simulink model "KUKA_EE_Controller_v4"  (R2021b)
settings: Solver=ode4  StartTime=0.0  StopTime=100  FixedStep=0.01  RelTol=1e-3
InitFcn:
  | %rho_0t=[0.29;0.29;0.29]; %m
  | %V_0t=[-0.001;-0.001;0];%[-0.0005;-0.0005;0];
  | %w_t=[0;0;-0.002];
  | 
  | 
  | %rho_0t=[0.3;0.3;0.2]; %m
  | %V_0t=[-0.001;-0.001;0];%[-0.0005;-0.0005;0];
  | %w_t=[0;0;-0.001];
values from neighbouring files (symbols this model uses):
  g_cm = zeros(4,4,n)    [Main.m]
  Im = zeros(3,3,n)    [Main.m]
  iota0 = eye(6,6)    [Internal_KUKA_Main.m]    (also in KUKA_Main.m; Main.m)
  K_d = 10*[1.3*eye(3) zeros(3);zeros(3) 0.8*eye(3)]    [Initiate_FQ.m]    (also in Internal_KUKA_Main.m = 200*[0.7*eye(3) zeros(3);zeros(3) 0.5*eye(3)]; KUKA_Main.m = [0.7*eye(3) zeros(3);zeros(3) 0.5*eye(3)]; Main.m = eye(6))
  K_i = 5*[0.1*eye(3) zeros(3);zeros(3) 0.01*eye(3)]    [Initiate_FQ.m]    (also in Internal_KUKA_Main.m = 200*[0.01*eye(3) zeros(3);zeros(3) 0.001*eye(3)]; KUKA_Main.m = [0.01*eye(3) zeros(3);zeros(3) 0.001*eye(3)]; Main.m = eye(6))
  K_p = 50*[0.1 0 0 0 0 0;0 0.1 0 0 0 0; 0 0 0.1 0 0 0; 0 0 0 0.01 0 0 ... (first row only)    [Initiate_FQ.m]    (also in Internal_KUKA_Main.m = 200*[0.1 0 0 0 0 0;0 0.1 0 0 0 0; 0 0 0.1 0 0 0; 0 0 0 0.01 ; KUKA_Main.m = [0.1 0 0 0 0 0;0 0.1 0 0 0 0; 0 0 0.1 0 0 0; 0 0 0 0.01 0 0; Main.m = eye(6))
  K_w = 20*eye(7)    [Initiate_FQ.m]
  K_wd = 1*eye(7)    [Initiate_FQ.m]
  M0 = M_temp.M0.data(:,:,1)    [Initiate_FQ.m]    (also in Internal_KUKA_Main.m; KUKA_Main.m; Main.m = simplify(transpose(robot.vehicle.iota_0)*robot.vehicle.M_fra)
  m0 = robot.Bodies{1,n+1}.Mass    [Internal_KUKA_Main.m]    (also in KUKA_Main.m; Main.m = 100)
  M0m = M_temp.M0m.data(:,:,1)    [Initiate_FQ.m]    (also in Internal_KUKA_Main.m; KUKA_Main.m; Main.m = simplify(transpose(robot.vehicle.iota_0)*transpose(Lm0)*diag)
  M_t = [eye(3)*mt zeros(3); zeros(3) eye(3)*0.416667]    [Initiate_FQ.m]    (also in Internal_KUKA_Main.m = [eye(3)*mt zeros(3); zeros(3) eye(3)*80]; KUKA_Main.m = [eye(3)*mt zeros(3); zeros(3) eye(3)*80]; Main.m = [eye(3)*mt zeros(3); zeros(3) eye(3)*416.667])
  Mm = simplify(transpose(Xi_m)*transpose(Lm)*diagM*Lm*Xi_m)    [Internal_KUKA_Main.m]    (also in KUKA_Main.m; Main.m)
  mm = zeros(1,n)    [Internal_KUKA_Main.m]    (also in KUKA_Main.m; Main.m = [2 2 0])
  mu = -10.*P0    [Initiate_FQ.m]    (also in Internal_KUKA_Main.m = P; KUKA_Main.m = P; Main.m = zeros(6,1)')
  mu_t = -10.*M_t*[V_0t;w_t]    [Initiate_FQ.m]    (also in Internal_KUKA_Main.m = M_t*[V_0t;w_t]; KUKA_Main.m = M_t*[V_0t;w_t]; Main.m = zeros(6,1)')
  q_dot_m = 0.01*q_dot_m    [Initiate_FQ.m]    (also in Internal_KUKA_Main.m = [qdot1;qdot2;qdot3;qdot4;qdot5;qdot6;qdot7]; KUKA_Main.m = [qdot1;qdot2;qdot3;qdot4;qdot5;qdot6;qdot7]; Main.m = [0;0;0;0;0;0;0]; sendJointTorques.m = fread(t, 7, 'double'))
  q_m = [0.2;1.2;0.3;1.8;0.5;1.3;0.6]    [Initiate_FQ.m]    (also in Internal_KUKA_Main.m = [q_m1;q_m2;q_m3;q_m4;q_m5;q_m6;q_m7]; KUKA_Main.m = [q_m1;q_m2;q_m3;q_m4;q_m5;q_m6;q_m7]; Main.m = [0;0;0;0;0;0;0]; sendJointTorques.m = fread(t, 7, 'double'))
  rho_0t = [0;0;0.2]    [Initiate_FQ.m]    (also in Internal_KUKA_Main.m = [0.24;0.26;0.25]; KUKA_Main.m = [0.23;0.27;0.26])
  sc_size = 0    [Internal_KUKA_Main.m]    (also in KUKA_Main.m = 1)
  V_0t = -[-0.0005;-0.0005;0]    [Initiate_FQ.m]    (also in Internal_KUKA_Main.m = [-0.01;-0.01;0]; KUKA_Main.m = [-0.002;-0.002;0])
  V_I0 = 0.01*V_I0    [Initiate_FQ.m]    (also in Internal_KUKA_Main.m = [0;0;0;0;0;0]; KUKA_Main.m = [0;0;0;0;0;0]; Main.m = [0;0;0;0;0;0])
  X = [0 -x(3) x(2) ; x(3) 0 -x(1) ; -x(2) x(1) 0 ]    [skewsym.m]
  Xi_m = Xi_m(1:robot.n*6,1:robot.n)    [Internal_KUKA_Main.m]    (also in KUKA_Main.m; Main.m)
  Xi_m_matrix = zeros(6*n,n)    [Internal_KUKA_Main.m]    (also in KUKA_Main.m; Main.m)
undefined symbols (not defined in the file or in its folder): g_cm0, I0, Ie, m0_frak, m_diag, me, Y, Z
libraries: sm_lib x174, nesl_utility x172, robotcorelib x7
(part 8 of 8)

== matlab function KUKA_EE_Controller_v4/Inverse Dynamics3/C_hat1/AMA_partial ==
  data: q_m input; AMA_partial output; M0 input; A input; A_partial input; V input; M0_partial input
function AMA_partial = AMA_partial(q_m,M0,A,A_partial,V,M0_partial)
% Calculates the C_hat_m matrix from base pose and arm joint angles

n=length(q_m);
b=length(V);

% find the temp intermediate term
AMA_partial=zeros(n,n,n);
for i=1:n
    AMA_partial(1:n,1:n,i)=transpose(A_partial(1:end,1:end,i))*M0*A+transpose(A)*M0_partial(1:end,1:end,i)*A+transpose(A)*M0*A_partial(1:end,1:end,i); %calcualte the derivative of not-augmented arm mass matrix from equation 121 of TRO paper
end

== matlab function KUKA_EE_Controller_v4/Inverse Dynamics3/C_hat1/A_partial ==
  data: q_m input; A_partial output; M0 input; M0_partial input; M0m_partial input; M0m input; V input
function A_partial = A_partial(q_m,M0,M0_partial,M0m_partial,M0m,V)
% Calculates the C_hat_m matrix from base pose and arm joint angles

n=length(q_m);
b=length(V);

% Find partial of connection A to each joint angle
A_partial=zeros(b,n,n);

temp1=zeros(b,n);
temp2=zeros(b,n);
temp3=zeros(b,n);

for i=1:n
    temp1=M0\M0_partial(1:end,1:end,i);
    temp2=M0\M0m;
    temp3=M0\M0m_partial(1:end,1:end,i);
    A_partial(1:b,1:n,i)=-temp1*temp2+temp3; % Equation 122
end

== matlab function KUKA_EE_Controller_v4/Dynamic Parameters/ 1 ==
  data: q_m input; L0 output; Lm0 output; Lm output; Xi_m input
function [L0,Lm0,Lm] =L_calculator(q_m,Xi_m)
% Calculates the time-dependent L matrix
n=length(q_m);
L=zeros(6*(n+1),6*(n+1));
% Compute M_frak for ith body
% Calculate L matrix
for i=1:n+1
    for j=1:n+1
        if i>j
            Ad_temp=eye(6);
            for k=j:i-1
                Ad_temp=Adjoint(g_Matrix(-Xi_m(:,k),q_m(k)))*Ad_temp;
            end
            L(6*(i-1)+1:6*(i-1)+6,6*(j-1)+1:6*(j-1)+6)=Ad_temp;
        elseif i==j
            L(6*(i-1)+1:6*(i-1)+6,6*(j-1)+1:6*(j-1)+6)=eye(6);
        elseif i<j
            L(6*(i-1)+1:6*(i-1)+6,6*(j-1)+1:6*(j-1)+6)=zeros(6);
        end
    end
end

L0=L(1:6,1:6);
Lm0=L(7:end,1:6);
Lm=L(7:end,7:end);

end

== matlab function KUKA_EE_Controller_v4/Inverse Dynamics3/C_hat1/C_hat ==
  data: q_m input; Mm_hat_partial input; q_dot_m input; C_hat output
function C_hat = C_hat(q_m, Mm_hat_partial,q_dot_m)
% Calculates the C_hat_m matrix from base pose and arm joint angles

n=length(q_m);


% Calculate C_hat matrix
C_temp1=zeros(n,n);
C_temp2=zeros(n,n);
C_hat=zeros(n,n);
for i=1:n
    C_temp1=C_temp1+squeeze(Mm_hat_partial(1:n,1:n,i)).*q_dot_m(i); % nxn by scalar
    C_temp2(i,1:n)=0.5*transpose(q_dot_m)*squeeze(Mm_hat_partial(1:n,1:n,i)); %1xn by nxn 
end

C_hat=C_temp1-C_temp2;

== matlab function KUKA_EE_Controller_v4/Inverse Dynamics3/C_hat1/Lm_partials/Lm0partial ==
  data: q_m input; Lm0_partial output; Xi_m input; iota0 input
function Lm0_partial = Lm0_partial(q_m,Xi_m,iota0)
% Calculates the C_hat_m matrix from base pose and arm joint angles

n=length(q_m);

% Find partial of Lm to joint angles
Lm0_partial=zeros(6*n,6,n); % 6nx6xn
for i=1:n
    for j=1:n
        Lm0_partial(6*(j-1)+1:6*j,1:6,i)=Ad_partial(j,1,i,Xi_m,q_m,iota0); % equation 114 of TRO paper
    end
end

%%%%%%%%%%%%%%%%%%%%%%%%%%%%%%%%%%%%%%%%%%%%%%%%%%%%%%%%%%%%% MUST BE
%%%%%%%%%%%%%%%%%%%%%%%%%%%%%%%%%%%%%%%%%%%%%%%%%%%%%%%%%%%%% CHECKED

== matlab function KUKA_EE_Controller_v4/Inverse Dynamics3/C_hat1/Lm_partials/Lmpartial ==
  data: q_m input; Lm_partial output; Xi_m input; iota0 input
function Lm_partial  = Lm_partial(q_m,Xi_m,iota0)
% Calculates the C_hat_m matrix from base pose and arm joint angles

n=length(q_m);

% Find partial of Lm0 to joint angles
Lm_partial=zeros(6*n,6*n,n); % 6nx6xn
for i=1:n
    Lm_partial(:,:,i)=zeros(6*n,6*n);
    for j=2:n
        for k=2:n
            if j>i && i>=k
                Lm_partial(6*(j-1)+1:6*j,6*(k-2)+1:6*(k-1),i)=Ad_partial(j,k,i,Xi_m,q_m,iota0); % equation 81 of TRO paper
            elseif i==j && i>=k
                Lm_partial(6*(j-1)+1:6*j,6*(k-2)+1:6*(k-1),i)=Ad_partial(j,k,i,Xi_m,q_m,iota0); % equation 81 of TRO paper
            else
                Lm_partial(6*(j-1)+1:6*(j-1)+6,6*(k-2)+1:6*(k-2)+6,i)=zeros(6,6);
            end

        end
    end
end

== matlab function KUKA_EE_Controller_v4/Inverse Dynamics3/C_hat1/M_partials/ M0partial ==
  data: q_m input; M0_partial output; Lm0 input; V input; iota0 input; diag_Mm input; Lm0_partial input
function M0_partial = M0_partial(q_m,Lm0,V,iota0,diag_Mm,Lm0_partial)
% Calculates the C_hat_m matrix from base pose and arm joint angles

n=length(q_m);
b=length(V);

% Find partial of M0 to joint angles
M0_partial=zeros(b,b,n); %initiate
for i=1:n
    temp1=transpose(Lm0_partial(1:end,1:end,i))*diag_Mm*Lm0;
    temp2=transpose(Lm0)*diag_Mm*Lm0_partial(1:end,1:end,i);
    M0_partial(1:b,1:b,i)= iota0'*(temp1+temp2)*iota0; %6x6 %equation 117 of TRO
end

== matlab function KUKA_EE_Controller_v4/Inverse Dynamics3/C_hat1/M_partials/M0mpartial ==
  data: q_m input; M0m_partial output; V input; Lm input; Lm0 input; iota0 input; diag_Mm input; Lm0_partial input; Lm_partial input; Xi_m_matrix input
function M0m_partial = M0m_partial(q_m,V,Lm,Lm0,iota0,diag_Mm,Lm0_partial,Lm_partial, Xi_m_matrix)
% Calculates the C_hat_m matrix from base pose and arm joint angles

n=length(q_m);
b=length(V);

% Find partial of M0m to joint angles
M0m_partial=zeros(b,n,n);
for i=1:n
    temp1=transpose(Lm0_partial(1:end,1:end,i))*diag_Mm*Lm;
    temp2=transpose(Lm0)*diag_Mm*Lm_partial(1:end,1:end,i);
    M0m_partial(1:b,1:n,i)= iota0'*(temp1+temp2)*Xi_m_matrix; % equation 118 of TRO paper
end

== matlab function KUKA_EE_Controller_v4/Inverse Dynamics3/C_hat1/M_partials/Mmpartial ==
  data: q_m input; Mm_partial output; Xi_m_matrix input; Lm input; diag_Mm input; Lm_partial input
function Mm_partial = Mm_partial(q_m,Xi_m_matrix,Lm,diag_Mm,Lm_partial)
% Calculates the C_hat_m matrix from base pose and arm joint angles

n=length(q_m);

% find the non-generalized arm mass matrix'x derivative to joint angles
Mm_partial=zeros(n,n,n);
for i=1:n
    temp=   transpose(Lm_partial(1:6*n,1:6*n,i))*diag_Mm*Lm  +   transpose(Lm)*diag_Mm*Lm_partial(1:6*n,1:6*n,i);
    Mm_partial(1:n,1:n,i)=transpose(Xi_m_matrix)*temp*Xi_m_matrix; %calcualte the derivative of not-augmented arm mass matrix from equation 120 of TRO paper
end

== matlab function KUKA_EE_Controller_v4/Inverse Dynamics3/C_hat1/Mm_hat_partial ==
  data: q_m input; AMA_partial input; Mm_hat_partial output; Mm_partial input
function Mm_hat_partial = Mm_hat_partial(q_m, AMA_partial, Mm_partial)
% Calculates the C_hat_m matrix from base pose and arm joint angles

n=length(q_m);

% find the generalized arm mass matrix'x derivative to joint angles
Mm_hat_partial=zeros(n,n,n);
for i=1:n
    Mm_hat_partial(1:n,1:n,i)=Mm_partial(1:n,1:n,i)-AMA_partial(1:n,1:n,i); %calcualte the derivative of augmented arm mass matrix from equation 119 of TRO paper
end

== matlab function KUKA_EE_Controller_v4/Inverse Dynamics3/N_hat1/N_hat ==
  data: N_hat_temp output; q_m input; q_dot_m input; A input; V input; P input; M0_partial input; A_partial input; iota0 input; M0 input
function N_hat_temp = N_hat(q_m,q_dot_m,A,V,P,M0_partial, A_partial, iota0, M0)
% Calculates the N_hat_m matrix from base pose and arm joint angles

n=length(q_m);
b=length(V);

%Form N_hat from equation 19 of ACC paper
N_temp1=zeros(n,b); N_temp2=zeros(n,b); N_temp3=zeros(n,b);

for i=1:n
    N_temp1=N_temp1+transpose(squeeze(A_partial(1:b,1:n,i)).*q_dot_m(i)); % transpose of (bxn times 1x1) 
    N_temp2(i,1:b)=transpose(q_dot_m)*transpose(squeeze(A_partial(1:b,1:n,i))); %1xn times nxb
    N_temp3(i,1:b)=0.5*transpose(P)*(M0\M0_partial(1:end,1:end,i))*inv(M0); % 1xb times bxb
end

N_hat_temp=transpose(A)*transpose(adjoint_low(V,iota0))-N_temp1+N_temp2+N_temp3;

== matlab function KUKA_EE_Controller_v4/Space Manipulator2/Q2q ==
  data: Q input; qm output
function qm = Q2q(Q)

qm=quat2eul(Q','XYZ')';

== matlab function KUKA_EE_Controller_v4/Controller/Velocity_error ==
  data: g_I0 input; V_Ie input; U_ff output; V_It input; V_It_dot input
function U_ff = U_ff(g_I0, V_Ie,V_It, V_It_dot)

U_ff=adjoint_low(Adjoint(g_I0)*V_Ie)*Adjoint(inv(g_I0))*V_It+Adjoint(inv(g_I0))*V_It_dot;

== matlab function KUKA_EE_Controller_v4/Space Manipulator2/Q2q1 ==
  data: Q input; qm output
function qm = Q2q(Q)

qm=quat2eul(Q','XYZ')';

== matlab function KUKA_EE_Controller_v4/Inverse Dynamics3/A_dot ==
  data: A_partial input; q_m input; A_dot output
function A_dot = fcn(A_partial, q_m)
n=length(q_m);

A_dot=zeros(6,n);
for i=1:n
    A_dot=A_dot+A_partial(:,:,i).*q_m(i);
end

== matlab function KUKA_EE_Controller_v4/Inverse Dynamics3/C_hat/AMA_partial ==
  data: q_m input; AMA_partial output; M0 input; A input; A_partial input; V input; M0_partial input
function AMA_partial = AMA_partial(q_m,M0,A,A_partial,V,M0_partial)
% Calculates the C_hat_m matrix from base pose and arm joint angles

n=length(q_m);
b=length(V);

% find the temp intermediate term
AMA_partial=zeros(n,n,n);
for i=1:n
    AMA_partial(1:n,1:n,i)=transpose(A_partial(1:end,1:end,i))*M0*A+transpose(A)*M0_partial(1:end,1:end,i)*A+transpose(A)*M0*A_partial(1:end,1:end,i); %calcualte the derivative of not-augmented arm mass matrix from equation 121 of TRO paper
end

== matlab function KUKA_EE_Controller_v4/Inverse Dynamics3/C_hat/A_partial ==
  data: q_m input; A_partial output; M0 input; M0_partial input; M0m_partial input; M0m input; V input
function A_partial = A_partial(q_m,M0,M0_partial,M0m_partial,M0m,V)
% Calculates the C_hat_m matrix from base pose and arm joint angles

n=length(q_m);
b=length(V);

% Find partial of connection A to each joint angle
A_partial=zeros(b,n,n);

temp1=zeros(b,n);
temp2=zeros(b,n);
temp3=zeros(b,n);

for i=1:n
    temp1=M0\(M0_partial(:,:,i));
    temp2=M0\M0m;
    temp3=M0\(M0m_partial(:,:,i));
    A_partial(1:b,1:n,i)=-temp1*temp2+temp3; % Equation 122
end

== matlab function KUKA_EE_Controller_v4/Inverse Dynamics3/C_hat/C_hat1 ==
  data: q_m input; Mm_hat_partial input; q_dot_m input; C_hat output
function C_hat = C_hat(q_m, Mm_hat_partial,q_dot_m)
% Calculates the C_hat_m matrix from base pose and arm joint angles

n=length(q_m);


% Calculate C_hat matrix
C_temp1=zeros(n,n);
C_temp2=zeros(n,n);
C_hat=zeros(n,n);
for i=1:n
    C_temp1=C_temp1+squeeze(Mm_hat_partial(1:n,1:n,i)).*q_dot_m(i); % nxn by scalar
    C_temp2(i,1:n)=0.5*transpose(q_dot_m)*squeeze(Mm_hat_partial(1:n,1:n,i)); %1xn by nxn 
end

C_hat=C_temp1-C_temp2;

== matlab function KUKA_EE_Controller_v4/Inverse Dynamics3/C_hat/Lm_partials/Lm0partial ==
  data: q_m input; Lm0_partial output; Xi_m input; iota0 input
function Lm0_partial = Lm0_partial(q_m,Xi_m,iota0)
% Calculates the C_hat_m matrix from base pose and arm joint angles

n=length(q_m);

% Find partial of Lm to joint angles
Lm0_partial=zeros(6*n,6,n); % 6nx6xn
for i=1:n
    for j=1:n
        Lm0_partial(6*(j-1)+1:6*j,1:6,i)=Ad_partial(j,1,i,Xi_m,q_m,iota0); % equation 114 of TRO paper
    end
end

%%%%%%%%%%%%%%%%%%%%%%%%%%%%%%%%%%%%%%%%%%%%%%%%%%%%%%%%%%%%% MUST BE
%%%%%%%%%%%%%%%%%%%%%%%%%%%%%%%%%%%%%%%%%%%%%%%%%%%%%%%%%%%%% CHECKED

== matlab function KUKA_EE_Controller_v4/Inverse Dynamics3/C_hat/Lm_partials/Lmpartial ==
  data: q_m input; Lm_partial output; Xi_m input; iota0 input
function Lm_partial  = Lm_partial(q_m,Xi_m,iota0)
% Calculates the C_hat_m matrix from base pose and arm joint angles

n=length(q_m);

% Find partial of Lm0 to joint angles
Lm_partial=zeros(6*n,6*n,n); % 6nx6xn
for i=1:n
    Lm_partial(:,:,i)=zeros(6*n,6*n);
    for j=2:n
        for k=2:n
            if j>i && i>=k
                Lm_partial(6*(j-1)+1:6*j,6*(k-2)+1:6*(k-1),i)=Ad_partial(j,k,i,Xi_m,q_m,iota0); % equation 81 of TRO paper
            elseif i==j && i>=k
                Lm_partial(6*(j-1)+1:6*j,6*(k-2)+1:6*(k-1),i)=Ad_partial(j,k,i,Xi_m,q_m,iota0); % equation 81 of TRO paper
            else
                Lm_partial(6*(j-1)+1:6*(j-1)+6,6*(k-2)+1:6*(k-2)+6,i)=zeros(6,6);
            end

        end
    end
end

== matlab function KUKA_EE_Controller_v4/Inverse Dynamics3/C_hat/M_partials/ M0partial ==
  data: q_m input; M0_partial output; Lm0 input; V input; iota0 input; diag_Mm input; Lm0_partial input
function M0_partial = M0_partial(q_m,Lm0,V,iota0,diag_Mm,Lm0_partial)
% Calculates the C_hat_m matrix from base pose and arm joint angles

n=length(q_m);
b=length(V);

% Find partial of M0 to joint angles
M0_partial=zeros(b,b,n); %initiate
for i=1:n
    temp1=transpose(Lm0_partial(1:end,1:end,i))*diag_Mm*Lm0;
    temp2=transpose(Lm0)*diag_Mm*Lm0_partial(1:end,1:end,i);
    M0_partial(1:b,1:b,i)= iota0'*(temp1+temp2)*iota0; %6x6 %equation 117 of TRO
end

== matlab function KUKA_EE_Controller_v4/Inverse Dynamics3/C_hat/M_partials/M0mpartial ==
  data: q_m input; M0m_partial output; V input; Lm input; Lm0 input; iota0 input; diag_Mm input; Lm0_partial input; Lm_partial input; Xi_m_matrix input
function M0m_partial = M0m_partial(q_m,V,Lm,Lm0,iota0,diag_Mm,Lm0_partial,Lm_partial, Xi_m_matrix)
% Calculates the C_hat_m matrix from base pose and arm joint angles

n=length(q_m);
b=length(V);

% Find partial of M0m to joint angles
M0m_partial=zeros(b,n,n);
for i=1:n
    temp1=transpose(Lm0_partial(1:end,1:end,i))*diag_Mm*Lm;
    temp2=transpose(Lm0)*diag_Mm*Lm_partial(1:end,1:end,i);
    M0m_partial(1:b,1:n,i)= iota0'*(temp1+temp2)*Xi_m_matrix; % equation 118 of TRO paper
end

== matlab function KUKA_EE_Controller_v4/Inverse Dynamics3/C_hat/M_partials/Mmpartial ==
  data: q_m input; Mm_partial output; Xi_m_matrix input; Lm input; diag_Mm input; Lm_partial input
function Mm_partial = Mm_partial(q_m,Xi_m_matrix,Lm,diag_Mm,Lm_partial)
% Calculates the C_hat_m matrix from base pose and arm joint angles

n=length(q_m);

% find the non-generalized arm mass matrix'x derivative to joint angles
Mm_partial=zeros(n,n,n);
for i=1:n
    temp=   transpose(Lm_partial(1:6*n,1:6*n,i))*diag_Mm*Lm  +   transpose(Lm)*diag_Mm*Lm_partial(1:6*n,1:6*n,i);
    Mm_partial(1:n,1:n,i)=transpose(Xi_m_matrix)*temp*Xi_m_matrix; %calcualte the derivative of not-augmented arm mass matrix from equation 120 of TRO paper
end

== matlab function KUKA_EE_Controller_v4/Controller/gradient_of_Eg ==
  data: g_te input; Nabla_Eg output
function Nabla_Eg = fcn(g_te)

% Calculate the gradient of the Pose Error Function
p_te=g_te(1:3,4);
R_te=g_te(1:3,1:3);

temp=0.5*(R_te-transpose(R_te));

R_temp=vee3(temp);

Nabla_Eg=[p_te;R_temp];

== matlab function KUKA_EE_Controller_v4/Inverse Dynamics3/C_hat/Mm_hat_partial ==
  data: q_m input; AMA_partial input; Mm_hat_partial output; Mm_partial input
function Mm_hat_partial = Mm_hat_partial(q_m, AMA_partial, Mm_partial)
% Calculates the C_hat_m matrix from base pose and arm joint angles

n=length(q_m);

% find the generalized arm mass matrix'x derivative to joint angles
Mm_hat_partial=zeros(n,n,n);
for i=1:n
    Mm_hat_partial(1:n,1:n,i)=Mm_partial(1:n,1:n,i)-AMA_partial(1:n,1:n,i); %calcualte the derivative of augmented arm mass matrix from equation 119 of TRO paper
end

== matlab function KUKA_EE_Controller_v4/Inverse Dynamics3/Inverse Dynamics/Ad_g_I0_dot ==
  data: g_I0 input; V_I0 input; Ad_g_I0_dot output
function Ad_g_I0_dot = Ad_g_I0_dot(g_I0,V_I0)
% Calculation of F_mu Eq 30 of paper
Ad_g_I0_dot=adjoint_low(V_I0)'*Adjoint(g_I0)';
% adjoint_low(V_I0)*transpose(Adjoint*(g_I0)))

== matlab function KUKA_EE_Controller_v4/Inverse Dynamics3/Inverse Dynamics/Ad_g_I0_dot1 ==
  data: V_t input; Ad_g_It_dot output; g_It input
function Ad_g_It_dot = Ad_g_It_dot(V_t,g_It)
% Calculation of F_mu Eq 30 of paper
Ad_g_It_dot=adjoint_low(V_t)'*Adjoint(g_It)';

== matlab function KUKA_EE_Controller_v4/Inverse Dynamics3/Inverse Dynamics/Ad_g_te_dot ==
  data: V_te input; Ad_g_te_dot output; g_te input
function Ad_g_te_dot = Ad_g_te_dot(V_te,g_te)
% Calculation of F_mu Eq 30 of paper
Ad_g_te_dot=-adjoint_low(V_te)/Adjoint(g_te);

== matlab function KUKA_EE_Controller_v4/Inverse Dynamics3/Inverse Dynamics/FU ==
  data: MmJcross input; F_U output
function F_U = F_U(MmJcross)
F_U=MmJcross;

== matlab function KUKA_EE_Controller_v4/Inverse Dynamics3/Inverse Dynamics/Fm ==
  data: MmJcross input; F_m output; A_dot input; Cm_hat input
function F_m = F_m(MmJcross,A_dot,Cm_hat)
% Calculation of F_mu Eq 30 of paper
F_m=MmJcross*(A_dot)+Cm_hat;

== matlab function KUKA_EE_Controller_v4/Inverse Dynamics3/Inverse Dynamics/Fmu ==
  data: MmJcross input; M0 input; M_0_dot input; g_I0 input; F_mu output; Ad_g_I0_dot input
function F_mu = F_mu(MmJcross,M0,M_0_dot,g_I0,Ad_g_I0_dot)
% Calculation of F_mu Eq 30 of paper
F_mu=-MmJcross*(M0\M_0_dot*inv(M0)*transpose(Adjoint(g_I0))+ ...
    M0\Ad_g_I0_dot);

== matlab function KUKA_EE_Controller_v4/Inverse Dynamics3/Inverse Dynamics/Inverse Dynamics ==
  data: F_mu output; F_t output; F_m output
function [F_mu,F_t,F_m] = fcn()


% n=length(q_m);

%Calculate Mass Matrix block components
% [ M0m Mm]=Mass_Matrix(q_m,Xi_m);

% A=inverse(M0)*M0m; % Mechanical Connection
% Mm_hat=Mm-transpose(A)*M0*A; %augmented manipulator mass matrix
% V=inverse(M0)*(mu-transpose(A)*q_dot_m); %Spacecraft Velocity

% The augmented Jacobian
% J_aug = J_em-J_e0*A;

% for i=1:n
%     for j=1:n
%         Cm_hat=
%     end
% end 

% Find A_dot thru finding partial of connection A to each joint angle
% A_partial=zeros(6,n,n);
% A_dot=zeros(6,n);
% for i=1:n
%     A_partial(6,n,i)=inverse(M0)*M0_partial(1:6,1:6,i)*inverse(M0)*M0m+inverse(M0)*M0m_partial(6,n,i); % Equation 122
%     A_dot(6,n)=A_dot+A_partial(6,n,i).*q_dot_m(i);
% end


% inverse or moore-penrose inverse of the augmented J2 Jacobian matrix
% if rank(J_aug)==size(J2(1,:))
%     J_inv=inverse(J2);
% else
%     J_inv=pinv(J2);
% end

% MJ_inv=-Mm_hat*J_cross;

% J_em_dot=J_em_dot;
% J_e0_dot=J_e0_dot;

% Form the eventual feedback transformation terms
% F_U=MmJcross; %done
% F_mu=MmJcross*(J_e0_dot*inverse(M0)*transpose(Adjoint*(g_I0))- ...
%     J_e0*inverse(M0)*M_0_dot*inverse(M0)*transpose(Adjoint*(g_I0))+ ...
%     J_e0*inverse(M0)*adjoint_low(inverse(M0*transpose(Adjoint(g_I0))*mu)-A*q_dot_m)); 
% F_t=MmJcross*();
% F_m=MmJcross*(J_em_dot-J_e0_dot*A-J_e0*A_dot)+Cm_hat;

== matlab function KUKA_EE_Controller_v4/Controller/Kinematics/g_te ==
  data: g_Ie input; g_It input; g_te output
function g_te = relative_pose(g_Ie, g_It)
% Calculates the relative pose of end-effector to target from the absolute
% poses of the end-effector and the target
g_te = inverse(g_It)*g_Ie;

== matlab function KUKA_EE_Controller_v4/Inverse Dynamics3/Inverse Dynamics/MATLAB Function3 ==
  data: MmJcross input; g_te input; F_t output; g_It input; Mt input; Ad_gte_dot input; Ad_gIt_dot input
function F_t = F_t(MmJcross,g_te,g_It,Mt,Ad_gte_dot,Ad_gIt_dot)
% Calculation of F_mu Eq 30 of paper
F_t=-MmJcross*(Ad_gte_dot/Mt*Adjoint(g_It)'+Adjoint(g_te)\(Mt\Ad_gIt_dot));

% F_t=MmJcross*(-adjoint_low(V_te)/Adjoint(g_te)/Adjoint(g_tt)/M_t/Adjoint(g_It)'+...
%     Adjoint()\); 

% J_e0_dot*inverse(M0)*transpose(Adjoint*(g_I0))- ...
%     J_e0*inverse(M0)*M_0_dot*inverse(M0)*transpose(Adjoint*(g_I0))+ ...
%     J_e0*inverse(M0)*adjoint_low(inverse(M0*transpose(Adjoint(g_I0))*mu)-A*q_dot_m)
%     Ad_g_te_dot

== matlab function KUKA_EE_Controller_v4/Inverse Dynamics3/Inverse Dynamics/MmJcross ==
  data: Mm_hat input; MmJcross output; A input
function MmJcross = MmJcross(Mm_hat, A)

JJ=-A;

% MmJcross = Mm_hat*pinv(JJ);
MmJcross = Mm_hat*pinv(JJ);%,10^(-3)

== matlab function KUKA_EE_Controller_v4/Inverse Dynamics3/Inverse Dynamics/Mm_hat ==
  data: M0 input; Mm_hat output; Mm input; A input
function Mm_hat = Mm_hat(M0,Mm,A)

Mm_hat=Mm-A'*M0*A;

== matlab function KUKA_EE_Controller_v4/Inverse Dynamics3/M0_dot ==
  data: M0_partial input; q_m input; M0_dot output
function M0_dot = fcn(M0_partial, q_m)
n=length(q_m);

M0_dot=zeros(6,6);
for i=1:n
    M0_dot=M0_dot+M0_partial(:,:,i).*q_m(i);
end

== matlab function KUKA_EE_Controller_v4/Inverse Dynamics3/N_hat/N_hat ==
  data: N_hat_temp output; q_m input; q_dot_m input; A input; V input; P input; M0_partial input; A_partial input; iota0 input; M0 input
function N_hat_temp = N_hat(q_m,q_dot_m,A,V,P,M0_partial, A_partial, iota0, M0)
% Calculates the N_hat_m matrix from base pose and arm joint angles

n=length(q_m);
b=length(V);

%Form N_hat from equation 19 of ACC paper
N_temp1=zeros(n,b); N_temp2=zeros(n,b); N_temp3=zeros(n,b);

for i=1:n
    N_temp1=N_temp1+transpose(squeeze(A_partial(1:b,1:n,i)).*q_dot_m(i)); % transpose of (bxn times 1x1) 
    N_temp2(i,1:b)=transpose(q_dot_m)*transpose(squeeze(A_partial(1:b,1:n,i))); %1xn times nxb
    N_temp3(i,1:b)=0.5*transpose(P)*(-M0\M0_partial(1:end,1:end,i)/M0); % 1xb times bxb
end

N_hat_temp=transpose(A)*transpose(adjoint_low(V,iota0))-N_temp1+N_temp2+N_temp3;

== matlab function KUKA_EE_Controller_v4/MATLAB Function ==
  data: A input; wt output
function wt = fcn(A)

J=-A;
% SVD=svd(J);

% minSVD=min(SVD);
% maxSVD=max(SVD);

wt=sqrt(det(J*J'));

% y = minSVD/maxSVD;

== matlab function KUKA_EE_Controller_v4/Controller/Kinematics/Pose Error Function ==
  data: g_te input; E_g output
function E_g = pose_Error_function(g_te)
% Calculates the pose Error function from the relative pose of end-effector to target
R_te=g_te(1:3,1:3);
p_te=g_te(1:3,4);

temp_R=eye(3)-R_te;
temp_R=0.5*trace(temp_R);

temp_p=0.5*transpose(p_te)*p_te;
E_g =temp_R+temp_p;

== matlab function KUKA_EE_Controller_v4/Controller/Kinematics/Velocity_error ==
  data: g_I0 input; V_Ie input; V_e output; V_It input
function V_e = Velocity_Error_function(g_I0, V_Ie,V_It)
% Calculates the Velocity Error function from the momentums of chaser and
% target and the joint velocities

V_te_I=V_Ie-V_It;%Adjoint(inv(g_I0))*
V_te=Adjoint(inv(g_I0))*V_te_I;
V_e=V_te;

== matlab function KUKA_EE_Controller_v4/Jacobian ==
  data: q input; J output; Xi input; iota0 input
function J = fcn(q,Xi,iota0)

for i=1:n
    Ad_temp=eye(6);
    for j=1:i
        Ad_temp=Ad_temp*Adjoint(Xi(:,i),q(i));
    end
    J=[iota0 Xi(:,1) ]
end
y = u;

== matlab function KUKA_EE_Controller_v4/Controller/MATLAB Function ==
  data: fw input; fw_scaled output
function fw_scaled = fcn(fw)

norm_fw=norm(fw);
fw_scaled = exp(norm_fw).*fw;

== matlab function KUKA_EE_Controller_v4/MATLAB Function1 ==
  data: J input; wt output
function wt = fcn(J)

% SVD=svd(J);

% minSVD=min(SVD);
% maxSVD=max(SVD);

wt=sqrt(det(J*J'));

% y = minSVD/maxSVD;

== matlab function KUKA_EE_Controller_v4/Controller/nullspace_mapping ==
  data: Mm input; A input; fw output; grad_w input
function fw =null_space(Mm,A, grad_w)

% temp=A/Mm;
temp=null(A);
m=length(temp(1,:));
null_space=zeros(7,m);
for i=1:m
    null_space(:,i)=Mm*temp(:,i);
end
fw=zeros(7,1);
for i=1:m
    fw =fw+ dot(grad_w, null_space(:,i)) / norm(null_space(:,i))^2 * null_space(:,i);
end
